simulink model "L12AcutatorModel"  (R2014a)
settings: Solver=ode45  StartTime=0.0  StopTime=30.0  RelTol=1e-3
undefined symbols (not defined in the file): K_L12_Force, K_PWM, Mar, Ra_L12
settings Model: Creator=oberstare  LastModifiedBy=oberstare

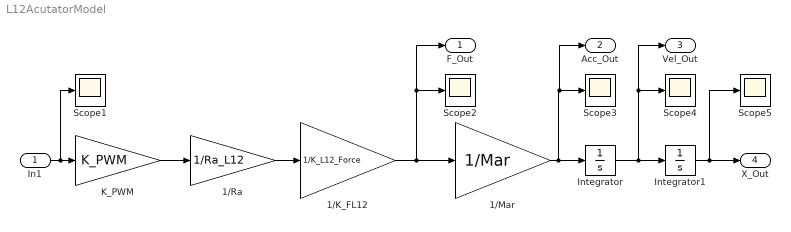
== system L12AcutatorModel ==
  In1 : Inport
  1/K_FL12 : Gain  Gain=1/K_L12_Force
  1/Mar : Gain  Gain=1/Mar
  1/Ra : Gain  Gain=1/Ra_L12
  Integrator : Integrator
  Integrator1 : Integrator
  K_PWM : Gain  Gain=K_PWM
  Scope{1..5} (5 alike) : Scope
      Scope1 settings: AttributesFormatString=%<ShowName>
      Scope2 settings: TimeRange=12  YMin=-1.59375  YMax=2.40625
      Scope3 settings: SaveName=ScopeData4
      Scope4 settings: SaveName=ScopeData2
      Scope5 settings: SaveName=ScopeData3
  F_Out : Outport
  Acc_Out : Outport  Port=2
  Vel_Out : Outport  Port=3
  X_Out : Outport  Port=4
  wires:
  Integrator/1 -> Vel_Out/1, Scope4/1, Integrator1/1
  K_PWM/1 -> 1/Ra/1
  1/Ra/1 -> 1/K_FL12/1
  1/K_FL12/1 -> F_Out/1, Scope2/1, 1/Mar/1
  Integrator1/1 -> Scope5/1, X_Out/1
  1/Mar/1 -> Acc_Out/1, Scope3/1, Integrator/1
  In1/1 -> Scope1/1, K_PWM/1
